simulink model "ESS_3P_2L_220kW_for_LS_Project"  (R2023b)
settings: Solver=VariableStepAuto  StartTime=0.0  StopTime=3  RelTol=1e-3
InitFcn:
  | %Initialization_for_ESS_3P_2L_220kW;
  | Initialization_for_ESS_3P_2L_220kW;
values from neighbouring files (symbols this model uses):
  C_grid = 54e-6    (= 5.4e-05)    [Initialization_for_ESS_3P_2L_220kW.m]    (also in Initialization_for_Testbench.m = 4.5e-05)
  Cdc = 180e-6    (= 0.00018)    [CurrentLoop.m]    (also in Initialization_for_ESS_3P_2L_220kW.m; Initialization_for_Testbench.m)
  Fnom_Grid = 50    [CurrentLoop.m]    (also in Initialization_for_ESS_3P_2L_220kW.m; Initialization_for_Testbench.m)
  Gain_for_ActiveDamping = 1    [Initialization_for_Testbench.m]
  Inom = Pnom/sqrt(3)/Unom_Grid    [CurrentLoop.m]    (also in Initialization_for_ESS_3P_2L_220kW.m; Initialization_for_Testbench.m)
  Ki_Edq = Kp_Edq*2*pi*10    (= 18.8495559215)    [Initialization_for_ESS_3P_2L_220kW.m]
  Ki_Idq = Kp_Idq*2*pi*10    (= 157.913670417)    [Initialization_for_ESS_3P_2L_220kW.m]    (also in Initialization_for_Testbench.m = 1.26330936334)
  Kp_Edq = 0.3    [Initialization_for_ESS_3P_2L_220kW.m]
  Kp_Idq = L_grid*2*pi*2000    (= 2.51327412287)    [Initialization_for_ESS_3P_2L_220kW.m]    (also in Initialization_for_Testbench.m = 2.0106192983)
  L_grid = 200e-6    (= 0.0002)    [Initialization_for_ESS_3P_2L_220kW.m]    (also in Initialization_for_Testbench.m)
  Pnom = 220e3    (= 220000)    [CurrentLoop.m]    (also in Initialization_for_ESS_3P_2L_220kW.m; Initialization_for_Testbench.m = 2500000)
  Ts_Control = 62.5e-6    (= 6.25e-05)    [CurrentLoop.m]    (also in Initialization_for_ESS_3P_2L_220kW.m; Initialization_for_Testbench.m = 0.0001)
  Ts_Power = 10e-7    (= 1e-06)    [Initialization_for_ESS_3P_2L_220kW.m]    (also in Initialization_for_Testbench.m)
  Udc_ref = 1500    [CurrentLoop.m]    (also in Initialization_for_ESS_3P_2L_220kW.m; Initialization_for_Testbench.m)
  Unom_Grid = 690    [CurrentLoop.m]    (also in Initialization_for_ESS_3P_2L_220kW.m; Initialization_for_Testbench.m)
  Unom_Phase = Unom_Grid/sqrt(3)    [CurrentLoop.m]    (also in Initialization_for_ESS_3P_2L_220kW.m; Initialization_for_Testbench.m)
undefined symbols (not defined in the file or in its folder): DiscIntNeverNeededParam, magnitude
libraries: LibraryForCodeGeneration x15, slpidlib x10, spsabctodq0Lib x7, spsAlphaBetaZerotoabcLib x6, simulink x5, spsThreePhaseVIMeasurementLib x4, spsVoltageMeasurementLib x4, eeGeneralControl x3, spsabctoAlphaBetaZeroLib x3, spsSeriesRLCBranchLib x3, spsThreePhaseSeriesRLCBranchLib x3, spsStairGeneratorLib x2
(part 2 of 2)

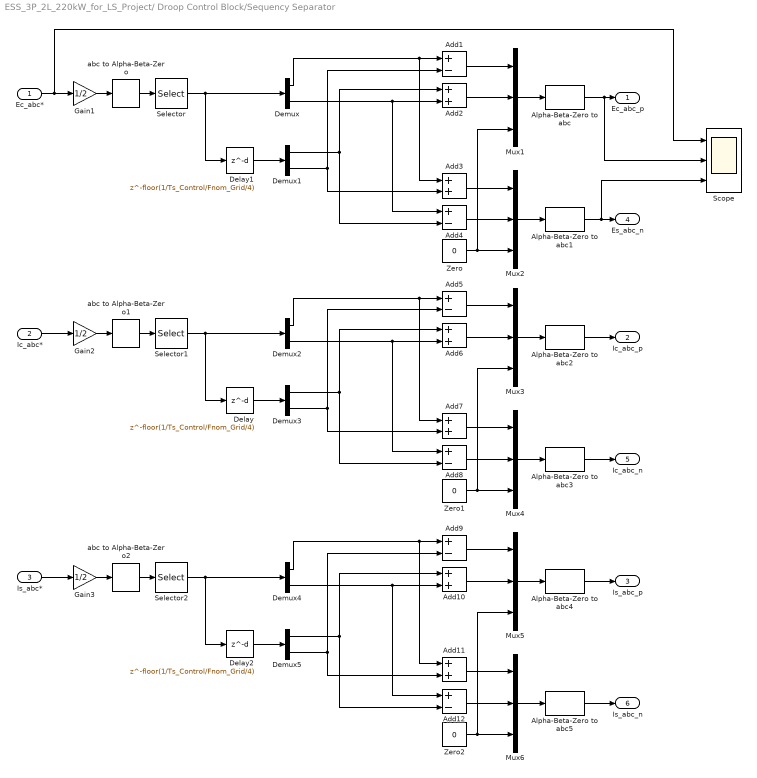
== system ESS_3P_2L_220kW_for_LS_Project/ Droop Control Block/Sequency Separator ==
  Ec_abc* : Inport
  " Ic_abc*" : Inport  Port=2
  Is_abc* : Inport  Port=3
  Add{1,4..5,8..9,12} (6 alike) : Sum  Inputs=+-
  Add{2..3,6..7,10..11} (6 alike) : Sum
  Alpha-Beta-Zero to abc{,1..5} (6 alike) : spsAlphaBetaZerotoabcLib/Alpha-Beta-Zero to abc
  Delay : Delay  DelayLength=floor(1/Ts_Control/Fnom_Grid/4)  SampleTime=Ts_Control
  Delay1 : Delay  DelayLength=floor(1/Ts_Control/Fnom_Grid/4)  SampleTime=Ts_Control
  Delay2 : Delay  DelayLength=floor(1/Ts_Control/Fnom_Grid/4)  SampleTime=Ts_Control
  Demux{,1..5} (6 alike) : Demux  Outputs=2
  Gain1 : Gain  Gain=1/2
  Gain2 : Gain  Gain=1/2
  Gain3 : Gain  Gain=1/2
  Mux{1..6} (6 alike) : Mux  Inputs=3
  Scope : Scope  NumInputPorts=3
  Selector : Selector  InputPortWidth=3  IndexOptions=Index vector (dialog)  Indices=[1 2]  OutputSizes=1
  Selector1 : Selector  InputPortWidth=3  IndexOptions=Index vector (dialog)  Indices=[1 2]  OutputSizes=1
  Selector2 : Selector  InputPortWidth=3  IndexOptions=Index vector (dialog)  Indices=[1 2]  OutputSizes=1
  Zero : Constant  Value=0  OutDataTypeStr=Inherit: Inherit via back propagation
  Zero1 : Constant  Value=0  OutDataTypeStr=Inherit: Inherit via back propagation
  Zero2 : Constant  Value=0  OutDataTypeStr=Inherit: Inherit via back propagation
  abc to Alpha-Beta-Zero : spsabctoAlphaBetaZeroLib/abc to Alpha-Beta-Zero
  abc to Alpha-Beta-Zero1 : spsabctoAlphaBetaZeroLib/abc to Alpha-Beta-Zero
  abc to Alpha-Beta-Zero2 : spsabctoAlphaBetaZeroLib/abc to Alpha-Beta-Zero
  Ec_abc_p : Outport
  Ic_abc_p : Outport  Port=2
  Is_abc_p : Outport  Port=3
  Es_abc_n : Outport  Port=4
  Ic_abc_n : Outport  Port=5
  Is_abc_n : Outport  Port=6
  wires:
  Is_abc*/1 -> Gain3/1
  Demux4/2 -> Add10/2, Add12/1
  Demux5/1 -> Add10/1, Add12/2
  Demux5/2 -> Add9/2, Add11/2
  Gain3/1 -> abc to Alpha-Beta-Zero2/1
  Demux4/1 -> Add9/1, Add11/1
  Delay2/1 -> Demux5/1
  Add12/1 -> Mux6/2
  Add11/1 -> Mux6/1
  Add10/1 -> Mux5/2
  Add9/1 -> Mux5/1
  Alpha-Beta-Zero to abc5/1 -> Is_abc_n/1
  Alpha-Beta-Zero to abc4/1 -> Is_abc_p/1
  Zero2/1 -> Mux6/3, Mux5/3
  Selector2/1 -> Demux4/1, Delay2/1
  abc to Alpha-Beta-Zero2/1 -> Selector2/1
  Mux5/1 -> Alpha-Beta-Zero to abc4/1
  Mux6/1 -> Alpha-Beta-Zero to abc5/1
  " Ic_abc*"/1 -> Gain2/1
  Mux4/1 -> Alpha-Beta-Zero to abc3/1
  Mux3/1 -> Alpha-Beta-Zero to abc2/1
  abc to Alpha-Beta-Zero1/1 -> Selector1/1
  Selector1/1 -> Delay/1, Demux2/1
  Zero1/1 -> Mux3/3, Mux4/3
  Alpha-Beta-Zero to abc2/1 -> Ic_abc_p/1
  Alpha-Beta-Zero to abc3/1 -> Ic_abc_n/1
  Add5/1 -> Mux3/1
  Add6/1 -> Mux3/2
  Add7/1 -> Mux4/1
  Add8/1 -> Mux4/2
  Delay/1 -> Demux3/1
  Demux2/1 -> Add7/1, Add5/1
  Gain2/1 -> abc to Alpha-Beta-Zero1/1
  Demux3/2 -> Add7/2, Add5/2
  Demux3/1 -> Add8/2, Add6/1
  Demux2/2 -> Add8/1, Add6/2
  Demux/2 -> Add2/2, Add4/1
  Demux1/1 -> Add2/1, Add4/2
  Demux1/2 -> Add1/2, Add3/2
  Gain1/1 -> abc to Alpha-Beta-Zero/1
  Demux/1 -> Add1/1, Add3/1
  Delay1/1 -> Demux1/1
  Add4/1 -> Mux2/2
  Add3/1 -> Mux2/1
  Add2/1 -> Mux1/2
  Add1/1 -> Mux1/1
  Alpha-Beta-Zero to abc1/1 -> Es_abc_n/1, Scope/3
  Alpha-Beta-Zero to abc/1 -> Ec_abc_p/1, Scope/2
  Zero/1 -> Mux2/3, Mux1/3
  Selector/1 -> Demux/1, Delay1/1
  abc to Alpha-Beta-Zero/1 -> Selector/1
  Mux1/1 -> Alpha-Beta-Zero to abc/1
  Mux2/1 -> Alpha-Beta-Zero to abc1/1
  Ec_abc*/1 -> Scope/1, Gain1/1

== system ESS_3P_2L_220kW_for_LS_Project/ Droop Control Block/Synchronous Phase ==
  Ec_abc : Inport
  Egrid_abc : Inport  Port=2
  En_SP : Inport  Port=3
  AND : Logic  IconShape=distinctive  AllPortsSameDT=off  OutDataTypeStr=boolean
  Abs : Abs  SaturateOnIntegerOverflow=off
  Abs1 : Abs  SaturateOnIntegerOverflow=off
  Compare To Constant : simulink/Logic and Bit Operations/Compare To Constant  relop=<=  const=3  OutDataTypeStr=boolean
  Compare To Constant1 : simulink/Logic and Bit Operations/Compare To Constant  relop=<=  const=100e-3  OutDataTypeStr=boolean
  Constant : Constant  Value=[0,0]
  Demux : Demux  Outputs=2
  Index Vector : MultiPortSwitch  DataPortOrder=Zero-based contiguous  Inputs=2  zeroidx=on  SaturateOnIntegerOverflow=off  InputSameDT=off
  Moving Average : eeGeneralControl/Moving Average  VariantControl=Variant1  LabelModeActiveChoice=Discrete  f=0.1*Fnom_Grid  x0=0  BufferSize=8192  Ts=Ts_Control
      settings: LibrarySourceBlock=ee_sl_lib/General Control/Moving Average
  Moving Average1 : eeGeneralControl/Moving Average  VariantControl=Variant1  LabelModeActiveChoice=Discrete  f=0.1*Fnom_Grid  x0=0  BufferSize=8192  Ts=Ts_Control
      settings: LibrarySourceBlock=ee_sl_lib/General Control/Moving Average
  Subsystem : Subsystem
  COM : Outport
  Delta_Es : Outport  Port=2
  wires:
  Moving Average/1 -> Compare To Constant/1
  Abs/1 -> Moving Average/1
  Moving Average1/1 -> Compare To Constant1/1
  Abs1/1 -> Moving Average1/1
  AND/1 -> COM/1
  Compare To Constant/1 -> AND/1
  Compare To Constant1/1 -> AND/2
  Subsystem/1(Delta_Es) -> Demux/1, Index Vector/3
  Egrid_abc/1 -> Subsystem/1(Es)
  Ec_abc/1 -> Subsystem/2(Ec)
  En_SP/1 -> Subsystem/Enable, Index Vector/1
  Demux/1 -> Abs/1
  Demux/2 -> Abs1/1
  Index Vector/1 -> Delta_Es/1
  Constant/1 -> Index Vector/2

== system ESS_3P_2L_220kW_for_LS_Project/ Droop Control Block/Udq2Uabc ==
  Udq_p : Inport
  Udq_n : Inport  Port=2
  wt : Inport  Port=3
  Add : Sum
  Gain2 : Gain  Gain=-1
  Mux1 : Mux  Inputs=2
  Mux2 : Mux  Inputs=2
  Saturation : Saturate  UpperLimit=1.15  LowerLimit=-1.15
  Scope : Scope  NumInputPorts=3
  Zero1 : Constant  Value=0  OutDataTypeStr=Inherit: Inherit via back propagation
  Zero2 : Constant  Value=0  OutDataTypeStr=Inherit: Inherit via back propagation
  dq0 to abc : spsdq0toabcLib/dq0 to abc  Alignment=Aligned with phase A axis
  dq0 to abc1 : spsdq0toabcLib/dq0 to abc  Alignment=Aligned with phase A axis
  Uabc : Outport
  wires:
  Saturation/1 -> Uabc/1
  Zero2/1 -> Mux1/2
  dq0 to abc/1 -> Add/1, Scope/1
  Add/1 -> Scope/3, Saturation/1
  Udq_n/1 -> Mux2/1
  Mux2/1 -> dq0 to abc1/1
  Udq_p/1 -> Mux1/1
  Mux1/1 -> dq0 to abc/1
  Zero1/1 -> Mux2/2
  Gain2/1 -> dq0 to abc1/2
  wt/1 -> dq0 to abc/2, Gain2/1
  dq0 to abc1/1 -> Add/2, Scope/2

== system ESS_3P_2L_220kW_for_LS_Project/ Droop Control Block/Voltage Conversion ==
  Phase-Phase : Inport
  Add : Sum  Inputs=+-
  Add1 : Sum
  Add2 : Sum  Inputs=--
  Demux : Demux  Outputs=3
  Gain : Gain  Gain=1/3
  Gain1 : Gain  Gain=2
  Gain2 : Gain  Gain=2
  Mux : Mux  Inputs=3
  Terminator : Terminator
  Phase-Ground : Outport
  wires:
  Demux/3 -> Terminator/1
  Gain2/1 -> Add2/2
  Gain1/1 -> Add1/1
  Demux/2 -> Add/1, Add1/2, Gain2/1
  Demux/1 -> Gain1/1, Add2/1, Add/2
  Add2/1 -> Mux/3
  Add1/1 -> Mux/1
  Add/1 -> Mux/2
  Mux/1 -> Phase-Ground/1
  Gain/1 -> Demux/1
  Phase-Phase/1 -> Gain/1

== system ESS_3P_2L_220kW_for_LS_Project/ Droop Control Block/Voltage Conversion1 ==
  Phase-Phase : Inport
  Add : Sum  Inputs=+-
  Add1 : Sum
  Add2 : Sum  Inputs=--
  Demux : Demux  Outputs=3
  Gain : Gain  Gain=1/3
  Gain1 : Gain  Gain=2
  Gain2 : Gain  Gain=2
  Mux : Mux  Inputs=3
  Terminator : Terminator
  Phase-Ground : Outport
  wires:
  Demux/3 -> Terminator/1
  Gain2/1 -> Add2/2
  Gain1/1 -> Add1/1
  Demux/2 -> Add/1, Add1/2, Gain2/1
  Demux/1 -> Gain1/1, Add2/1, Add/2
  Add2/1 -> Mux/3
  Add1/1 -> Mux/1
  Add/1 -> Mux/2
  Mux/1 -> Phase-Ground/1
  Gain/1 -> Demux/1
  Phase-Phase/1 -> Gain/1

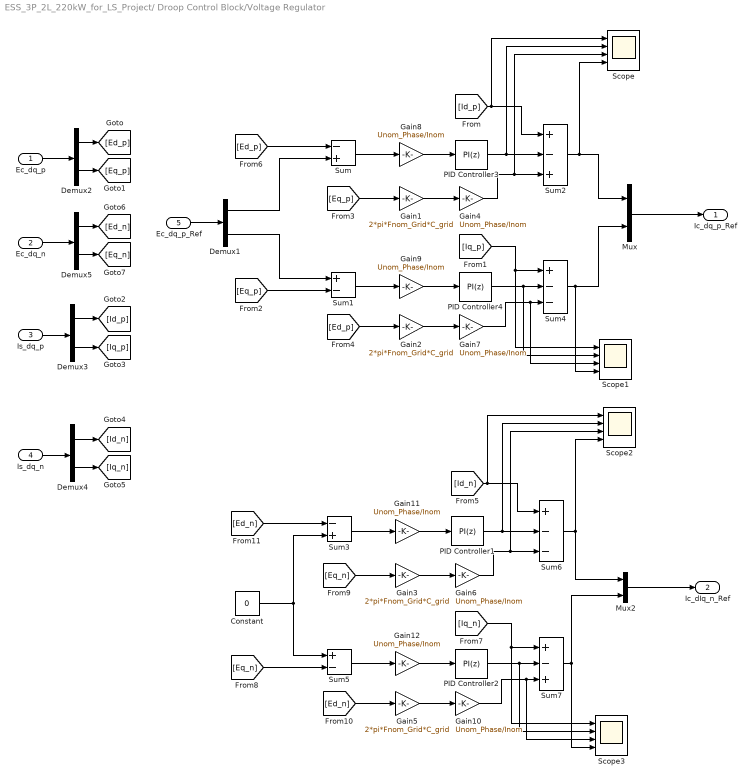
== system ESS_3P_2L_220kW_for_LS_Project/ Droop Control Block/Voltage Regulator ==
  Ec_dq_p : Inport
  Ec_dq_n : Inport  Port=2
  Is_dq_p : Inport  Port=3
  Is_dq_n : Inport  Port=4
  Ec_dq_p_Ref : Inport  Port=5  PortDimensions=2
  Constant : Constant  Value=0
  Demux{1..5} (5 alike) : Demux  Outputs=2
  Gain{1..3,5} (4 alike) : Gain  Gain=2*pi*Fnom_Grid*C_grid
  Gain{4,6..12} (8 alike) : Gain  Gain=Unom_Phase/Inom
  Mux : Mux  Inputs=2
  Mux2 : Mux  Inputs=2
  PID Controller{1..4} (4 alike) : slpidlib/PID Controller  Controller=PI  Form=Parallel  TimeDomain=Discrete-time  UseExternalTs=off  SampleTime=Ts_Control  IntegratorMethod=Forward Euler  FilterMethod=Forward Euler  ControllerParametersSource=internal  P=Kp_Edq  I=Ki_Edq  UseKiTs=off  D=0  N=100  UseFilter=on  TunerSelectOption=Transfer Function Based (PID Tuner App)  InitialConditionSource=internal  InitialConditionForIntegrator=0  InitialConditionForFilter=0  DifferentiatorICPrevScaledInput=0  ExternalReset=none  TrackingMode=off  Kt=1  LimitOutput=on  SatLimitsSource=internal  UpperSaturationLimit=2  LowerSaturationLimit=-2  LinearizeAsGain=on  AntiWindupMode=clamping  Kb=1  LimitIntegrator=off  UpperIntegratorSaturationLimit=inf  LowerIntegratorSaturationLimit=-inf  POutMin=[]  POutMax=[]  IOutMin=[]  IOutMax=[]  DOutMin=[]  DOutMax=[]  NOutMin=[]  NOutMax=[]  SumOutMin=[]  SumOutMax=[]  SaturationOutMin=[]  SaturationOutMax=[]  PParamMin=[]  PParamMax=[]  IParamMin=[]  IParamMax=[]  DParamMin=[]  DParamMax=[]  NParamMin=[]  NParamMax=[]  KbParamMin=[]  KbParamMax=[]  KtParamMin=[]  KtParamMax=[]  KbOutMin=[]  KbOutMax=[]  KtOutMin=[]  KtOutMax=[]  IntegratorOutMin=[]  IntegratorOutMax=[]  FilterOutMin=[]  FilterOutMax=[]  SumI1OutMin=[]  SumI1OutMax=[]  SumI2OutMin=[]  SumI2OutMax=[]  SumI3OutMin=[]  SumI3OutMax=[]  SumI4OutMin=[]  SumI4OutMax=[]  SumDOutMin=[]  SumDOutMax=[]  DifferentiatorOutMin=[]  DifferentiatorOutMax=[]  FilterDiffOutCoefMin=[]  FilterDiffOutCoefMax=[]  ReciprocalOutMin=[]  ReciprocalOutMax=[]  SumDenOutMin=[]  SumDenOutMax=[]  SumNumOutMin=[]  SumNumOutMax=[]  DivideOutMin=[]  DivideOutMax=[]  UdiffTsProdOutMin=[]  UdiffTsProdOutMax=[]  NTsProdOutMin=[]  NTsProdOutMax=[]  UintegralTsProdOutMin=[]  UintegralTsProdOutMax=[]  UngainTsProdOutMin=[]  UngainTsProdOutMax=[]  ClampingZeroOutDataTypeStr=Inherit: Inherit via back propagation  ClampingZeroOutMin=[]  ClampingZeroOutMax=[]  FilterDenConstantOutDataTypeStr=Inherit: Inherit via back propagation  FilterDenConstantOutMin=[]  FilterDenConstantOutMax=[]  PCopyOutDataTypeStr=Inherit: Inherit via back propagation  PCopyOutMin=[]  PCopyOutMax=[]  NCopyOutDataTypeStr=Inherit: Inherit via back propagation  NCopyOutMin=[]  NCopyOutMax=[]  IntegratorContinuousStateAttributes=''  IntegratorStateMustResolveToSignalObject=off  IntegratorRTWStateStorageClass=Auto  FilterContinuousStateAttributes=''  FilterStateMustResolveToSignalObject=off  FilterRTWStateStorageClass=Auto  ParallelPVariant=InternalParameters  IdealPVariant=Disabled  IVariant=InternalParameters  DVariant=Disabled  IntegratorVariant=Discrete  SatVariant=Enabled  AWVariant=DiscClampingParallel  PCopyVariant=Disabled  TRVariant=Disabled  FdbkBlocksVariant=Forward  IdealPFdbkVariant=Disabled  SatFdbkVariant=Disabled  DerivativeFilterVariant=Disabled  NVariant=Disabled  NCopyVariant=Disabled_SignalSpec  FilterICVariant=Disabled  IntegratorICVariant=InternalICs  ExternalResetVariant=Disabled  TRSumVariant=Passthrough  SumFdbkVariant=Disabled  SumVariant=Sum_PI  TsampFilterVariant=InternalTs  TsampNgainVariant=Passthrough  TsampIntegralVariant=Disabled_SignalSpec  ExternalSaturationOutDataTypeStr=Inherit: Same as second input
  Scope{,1..3} (4 alike) : Scope  NumInputPorts=4
  Sum : Sum  Inputs=-+  InputSameDT=on  SaturateOnIntegerOverflow=on  OutDataTypeStr=Inherit: Same as first input
  Sum1 : Sum  Inputs=+-  InputSameDT=on  SaturateOnIntegerOverflow=on  OutDataTypeStr=Inherit: Same as first input
  Sum2 : Sum  Inputs=+-+  InputSameDT=on  SaturateOnIntegerOverflow=on  OutDataTypeStr=Inherit: Same as first input
  Sum3 : Sum  Inputs=-+  InputSameDT=on  SaturateOnIntegerOverflow=on  OutDataTypeStr=Inherit: Same as first input
  Sum4 : Sum  Inputs=+--  InputSameDT=on  SaturateOnIntegerOverflow=on  OutDataTypeStr=Inherit: Same as first input
  Sum5 : Sum  Inputs=+-  InputSameDT=on  SaturateOnIntegerOverflow=on  OutDataTypeStr=Inherit: Same as first input
  Sum6 : Sum  Inputs=+--  InputSameDT=on  SaturateOnIntegerOverflow=on  OutDataTypeStr=Inherit: Same as first input
  Sum7 : Sum  Inputs=+-+  InputSameDT=on  SaturateOnIntegerOverflow=on  OutDataTypeStr=Inherit: Same as first input
  Ic_dq_p_Ref : Outport
  Ic_dIq_n_Ref : Outport  Port=2
  wires:
  Demux2/1 -> [Ed_p]
  [Ed_p] -> Gain2/1
  [Ed_p] -> Sum/1
  Sum2/1 -> Scope/4, Mux/1
  Gain8/1 -> PID Controller3/1
  Is_dq_p/1 -> Demux3/1
  Demux1/1 -> Sum/2
  Demux3/2 -> [Iq_p]
  Gain4/1 -> Scope/3, Sum2/3
  Demux1/2 -> Sum1/1
  Demux3/1 -> [Id_p]
  Sum4/1 -> Scope1/4, Mux/2
  [Eq_p] -> Sum1/2
  [Iq_p] -> Sum4/1, Scope1/1
  [Eq_p] -> Gain1/1
  Ec_dq_p/1 -> Demux2/1
  Sum1/1 -> Gain9/1
  Sum/1 -> Gain8/1
  Ec_dq_p_Ref/1 -> Demux1/1
  Gain1/1 -> Gain4/1
  Gain9/1 -> PID Controller4/1
  Gain7/1 -> Scope1/3, Sum4/3
  Gain2/1 -> Gain7/1
  PID Controller4/1 -> Scope1/2, Sum4/2
  PID Controller3/1 -> Scope/2, Sum2/2
  Demux2/2 -> [Eq_p]
  [Id_p] -> Scope/1, Sum2/1
  Mux/1 -> Ic_dq_p_Ref/1
  Demux4/2 -> [Iq_n]
  Demux4/1 -> [Id_n]
  Is_dq_n/1 -> Demux4/1
  Gain5/1 -> Gain10/1
  [Id_n] -> Scope2/1, Sum6/1
  PID Controller1/1 -> Scope2/2, Sum6/2
  PID Controller2/1 -> Scope3/2, Sum7/2
  Gain11/1 -> PID Controller1/1
  Sum3/1 -> Gain11/1
  Sum6/1 -> Mux2/1, Scope2/4
  Gain10/1 -> Scope3/3, Sum7/3
  [Iq_n] -> Sum7/1, Scope3/1
  Gain3/1 -> Gain6/1
  [Eq_n] -> Gain3/1
  [Eq_n] -> Sum5/2
  Sum5/1 -> Gain12/1
  Sum7/1 -> Mux2/2, Scope3/4
  Gain6/1 -> Scope2/3, Sum6/3
  [Ed_n] -> Sum3/1
  Gain12/1 -> PID Controller2/1
  [Ed_n] -> Gain5/1
  Constant/1 -> Sum5/1, Sum3/2
  Demux5/2 -> [Eq_n]
  Ec_dq_n/1 -> Demux5/1
  Demux5/1 -> [Ed_n]
  Mux2/1 -> Ic_dIq_n_Ref/1

== system ESS_3P_2L_220kW_for_LS_Project/ Droop Control Block/abc2dq_n ==
  Ec_abc_n : Inport
  "Ic_abc_n " : Inport  Port=2
  Is_abc_n : Inport  Port=3
  wt : Inport  Port=4
  Gain2 : Gain  Gain=-1
  Selector : Selector  InputPortWidth=3  IndexOptions=Index vector (dialog)  Indices=[1 2]  OutputSizes=1
  Selector1 : Selector  InputPortWidth=3  IndexOptions=Index vector (dialog)  Indices=[1 2]  OutputSizes=1
  Selector2 : Selector  InputPortWidth=3  IndexOptions=Index vector (dialog)  Indices=[1 2]  OutputSizes=1
  abc to dq0 : spsabctodq0Lib/abc to dq0  Alignment=Aligned with phase A axis
  abc to dq1 : spsabctodq0Lib/abc to dq0  Alignment=Aligned with phase A axis
  abc to dq2 : spsabctodq0Lib/abc to dq0  Alignment=Aligned with phase A axis
  Ec_dq_n : Outport
  Ic_dq_n : Outport  Port=2
  Is_dq_n : Outport  Port=3
  wires:
  Gain2/1 -> abc to dq0/2, abc to dq1/2, abc to dq2/2
  Is_abc_n/1 -> abc to dq2/1
  abc to dq2/1 -> Selector2/1
  Selector2/1 -> Is_dq_n/1
  wt/1 -> Gain2/1
  Ec_abc_n/1 -> abc to dq0/1
  "Ic_abc_n "/1 -> abc to dq1/1
  abc to dq1/1 -> Selector1/1
  abc to dq0/1 -> Selector/1
  Selector/1 -> Ec_dq_n/1
  Selector1/1 -> Ic_dq_n/1

== system ESS_3P_2L_220kW_for_LS_Project/ Droop Control Block/abc2dq_p ==
  Ec_abc_p : Inport
  "Ic_abc_p " : Inport  Port=2
  Is_abc_p : Inport  Port=3
  wt : Inport  Port=4
  Selector : Selector  InputPortWidth=3  IndexOptions=Index vector (dialog)  Indices=[1 2]  OutputSizes=1
  Selector1 : Selector  InputPortWidth=3  IndexOptions=Index vector (dialog)  Indices=[1 2]  OutputSizes=1
  Selector2 : Selector  InputPortWidth=3  IndexOptions=Index vector (dialog)  Indices=[1 2]  OutputSizes=1
  abc to dq0 : spsabctodq0Lib/abc to dq0  Alignment=Aligned with phase A axis
  abc to dq1 : spsabctodq0Lib/abc to dq0  Alignment=Aligned with phase A axis
  abc to dq2 : spsabctodq0Lib/abc to dq0  Alignment=Aligned with phase A axis
  Ec_dq_p : Outport
  Ic_dq_p : Outport  Port=2
  Is_dq_p : Outport  Port=3
  wires:
  abc to dq2/1 -> Selector2/1
  Selector2/1 -> Is_dq_p/1
  Is_abc_p/1 -> abc to dq2/1
  wt/1 -> abc to dq0/2, abc to dq1/2, abc to dq2/2
  Selector1/1 -> Ic_dq_p/1
  Selector/1 -> Ec_dq_p/1
  abc to dq0/1 -> Selector/1
  abc to dq1/1 -> Selector1/1
  "Ic_abc_p "/1 -> abc to dq1/1
  Ec_abc_p/1 -> abc to dq0/1

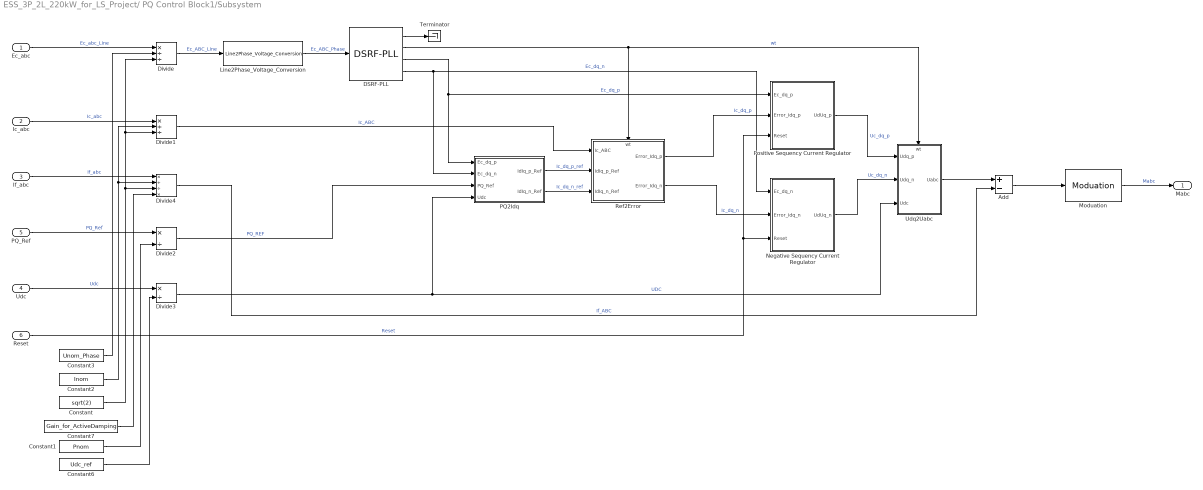
== system ESS_3P_2L_220kW_for_LS_Project/ PQ Control Block1/Subsystem ==
  Ec_abc : Inport  OutDataTypeStr=single  PortDimensions=3
  Ic_abc : Inport  Port=2  OutDataTypeStr=single  PortDimensions=3
  If_abc : Inport  Port=3  OutDataTypeStr=single  PortDimensions=3
  Udc : Inport  Port=4  OutDataTypeStr=single
  PQ_Ref : Inport  Port=5  OutDataTypeStr=single
  Reset : Inport  Port=6  OutDataTypeStr=boolean
  Add : Sum  Inputs=+-
  Constant : Constant  Value=sqrt(2)  OutDataTypeStr=Inherit: Inherit via back propagation  SampleTime=-1
  Constant1 : Constant  Value=Pnom  OutDataTypeStr=Inherit: Inherit via back propagation  SampleTime=-1
  Constant2 : Constant  Value=Inom  OutDataTypeStr=Inherit: Inherit via back propagation  SampleTime=-1
  Constant3 : Constant  Value=Unom_Phase  OutDataTypeStr=Inherit: Inherit via back propagation  SampleTime=-1
  Constant6 : Constant  Value=Udc_ref  OutDataTypeStr=Inherit: Inherit via back propagation  SampleTime=-1
  Constant7 : Constant  Value=Gain_for_ActiveDamping  OutDataTypeStr=Inherit: Inherit via back propagation  SampleTime=-1
  DSRF-PLL : LibraryForCodeGeneration/DSRF-PLL  Ts=Ts_Control  Wc=2*pi*50*0.707  Wf=2*pi*50  Kp=2*pi*25*2*0.707  Ki=power(2*pi*25,2)
  Divide : Product  Inputs=*//  OutDataTypeStr=single
  Divide1 : Product  Inputs=*//  OutDataTypeStr=single
  Divide2 : Product  Inputs=*/  OutDataTypeStr=single
  Divide3 : Product  Inputs=*/  OutDataTypeStr=single
  Divide4 : Product  Inputs=*//*  OutDataTypeStr=single
  Line2Phase_Voltage_Conversion : LibraryForCodeGeneration/Line2Phase_Voltage_Conversion  SystemSampleTime=-1  VariantActivationTime=update diagram  AllowFlexibleInterface=on  Latency=0  AutoFrameSizeCalculation=off
  Moduation : LibraryForCodeGeneration/Moduation  Modulation=SPWM
  Negative Sequency Current Regulator : Subsystem
  PQ2Idq : Subsystem  TreatAsAtomicUnit=on
  Positive Sequency Current Regulator : Subsystem
  Ref2Error : Subsystem
      settings: PortSchema="{\"entries\":[{\"content\":{\"sides\":[{\"content\":{\"connectorIds\":[\"In1\",\"In2\",\"In3\"]},\"type\":\"ConnectorPlacement.EquallySpacedRectSide\",\"uuid\":\"702c7fae-dbbb-427d-af19-afd468018ae6\"},{\"content\":{\"connectorIds\":[\"Out1\",\"Out2\"],\"side\":\"RIGHT\"},\"type\":\"ConnectorPlacement.EquallySpacedRectSide\",\"uuid\":\"d2ca5462-a446-46d8-bb73-1a455ffa959f\"},{\"content\":{\"connectorIds\":[\"In4\"],\"side\":\"TOP\"},\"type\":\"ConnectorPlacement.EquallySpacedRectSide\",\"uuid\":\"50bc6c44-424f-4342-960e-11540364fe97\"}]},\"type\":\"ConnectorPlacement.EquallySpacedConnector\",\"uuid\":\"f58cf64d-fe35-43f1-a031-7ee625a8bb1e\"}],\"packageUris\":[\"http://schema.mathworks.com/mf0/Connector/R2020b\"],\"version\":\"1.0\"}"
  Terminator : Terminator
  Udq2Uabc : Subsystem
      settings: PortSchema="{\"entries\":[{\"content\":{\"sides\":[{\"content\":{\"connectorIds\":[\"In1\",\"In2\",\"In3\"]},\"type\":\"ConnectorPlacement.EquallySpacedRectSide\",\"uuid\":\"009786f4-728c-4160-b9bf-eaf0b5a05101\"},{\"content\":{\"connectorIds\":[\"Out1\"],\"side\":\"RIGHT\"},\"type\":\"ConnectorPlacement.EquallySpacedRectSide\",\"uuid\":\"2a94367a-5c57-4632-9573-ab089470159a\"},{\"content\":{\"connectorIds\":[\"In4\"],\"side\":\"TOP\"},\"type\":\"ConnectorPlacement.EquallySpacedRectSide\",\"uuid\":\"6906365b-3187-4c4b-97cf-c9dec4c5ef7c\"}]},\"type\":\"ConnectorPlacement.EquallySpacedConnector\",\"uuid\":\"96ca8566-a266-405c-817a-b47b433d51ed\"}],\"packageUris\":[\"http://schema.mathworks.com/mf0/Connector/R2020b\"],\"version\":\"1.0\"}"
  Mabc : Outport  OutDataTypeStr=single  PortDimensions=3
  wires:
  Constant1/1 -> Divide2/2
  Negative Sequency Current Regulator/1(UdUq_n) -> Udq2Uabc/2(Udq_n)  "Uc_dq_n"
  Divide4/1 -> Add/2  "If_ABC"
  Udq2Uabc/1(Uabc) -> Add/1
  Constant6/1 -> Divide3/2
  Constant7/1 -> Divide4/4
  PQ_Ref/1 -> Divide2/1  "PQ_Ref"
  Add/1 -> Moduation/1
  DSRF-PLL/1 -> Terminator/1
  Moduation/1 -> Mabc/1  "Mabc"
  Reset/1 -> Positive Sequency Current Regulator/3(Reset), Negative Sequency Current Regulator/3(Reset)  "Reset"
  DSRF-PLL/2 -> Udq2Uabc/4(wt), Ref2Error/4(wt)  "wt"
  If_abc/1 -> Divide4/1  "If_abc"
  DSRF-PLL/4 -> PQ2Idq/2(Ec_dq_n), Negative Sequency Current Regulator/1(Ec_dq_n)  "Ec_dq_n"
  PQ2Idq/2(IdIq_n_Ref) -> Ref2Error/3(IdIq_n_Ref)  "Ic_dq_n_ref"
  Divide/1 -> Line2Phase_Voltage_Conversion/1  "Ec_ABC_Line"
  Udc/1 -> Divide3/1  "Udc"
  Constant/1 -> Divide4/3, Divide1/3, Divide/3
  Constant3/1 -> Divide/2
  Divide1/1 -> Ref2Error/1("Ic_ABC ")  "Ic_ABC"
  DSRF-PLL/3 -> Positive Sequency Current Regulator/1(Ec_dq_p), PQ2Idq/1(Ec_dq_p)  "Ec_dq_p"
  PQ2Idq/1(IdIq_p_Ref) -> Ref2Error/2("IdIq_p_Ref ")  "Ic_dq_p_ref"
  Positive Sequency Current Regulator/1(UdUq_p) -> Udq2Uabc/1(Udq_p)  "Uc_dq_p"
  Ref2Error/2(Error_Idq_n) -> Negative Sequency Current Regulator/2(Error_Idq_n)  "Ic_dq_n"
  Divide3/1 -> Udq2Uabc/3(Udc), PQ2Idq/4(Udc)  "UDC"
  Divide2/1 -> PQ2Idq/3(PQ_Ref)  "PQ_REF"
  Ic_abc/1 -> Divide1/1  "Ic_abc"
  Constant2/1 -> Divide4/2, Divide1/2
  Ref2Error/1(Error_Idq_p) -> Positive Sequency Current Regulator/2(Error_Idq_p)  "Ic_dq_p"
  Line2Phase_Voltage_Conversion/1 -> DSRF-PLL/1  "Ec_ABC_Phase"
  Ec_abc/1 -> Divide/1  "Ec_abc_Line"

== system ESS_3P_2L_220kW_for_LS_Project/ Droop Control Block/Synchronous Phase/Subsystem ==
  Es : Inport
  Ec : Inport  Port=2
  Enable : EnablePort  StatesWhenEnabling=reset
  Add1 : Sum  Inputs=-+
  Add2 : Sum  Inputs=+-
  Add3 : Sum  Inputs=-+
  Constant1 : Constant  Value=0
  Constant2 : Constant  Value=pi/2
  Constant3 : Constant
  Mux : Mux  Inputs=2
  PID Controller1 : slpidlib/PID Controller  Controller=PI  Form=Parallel  TimeDomain=Discrete-time  UseExternalTs=off  SampleTime=Ts_Control  IntegratorMethod=Forward Euler  FilterMethod=Forward Euler  ControllerParametersSource=internal  P=Kp_Edq*1  I=Kp_Edq*2*pi*0.01  UseKiTs=off  D=0  N=100  UseFilter=on  TunerSelectOption=Transfer Function Based (PID Tuner App)  InitialConditionSource=internal  InitialConditionForIntegrator=0  InitialConditionForFilter=0  DifferentiatorICPrevScaledInput=0  ExternalReset=none  TrackingMode=off  Kt=1  LimitOutput=on  SatLimitsSource=internal  UpperSaturationLimit=0.2  LowerSaturationLimit=-0.2  LinearizeAsGain=on  AntiWindupMode=clamping  Kb=1  LimitIntegrator=off  UpperIntegratorSaturationLimit=inf  LowerIntegratorSaturationLimit=-inf  POutMin=[]  POutMax=[]  IOutMin=[]  IOutMax=[]  DOutMin=[]  DOutMax=[]  NOutMin=[]  NOutMax=[]  SumOutMin=[]  SumOutMax=[]  SaturationOutMin=[]  SaturationOutMax=[]  PParamMin=[]  PParamMax=[]  IParamMin=[]  IParamMax=[]  DParamMin=[]  DParamMax=[]  NParamMin=[]  NParamMax=[]  KbParamMin=[]  KbParamMax=[]  KtParamMin=[]  KtParamMax=[]  KbOutMin=[]  KbOutMax=[]  KtOutMin=[]  KtOutMax=[]  IntegratorOutMin=[]  IntegratorOutMax=[]  FilterOutMin=[]  FilterOutMax=[]  SumI1OutMin=[]  SumI1OutMax=[]  SumI2OutMin=[]  SumI2OutMax=[]  SumI3OutMin=[]  SumI3OutMax=[]  SumI4OutMin=[]  SumI4OutMax=[]  SumDOutMin=[]  SumDOutMax=[]  DifferentiatorOutMin=[]  DifferentiatorOutMax=[]  FilterDiffOutCoefMin=[]  FilterDiffOutCoefMax=[]  ReciprocalOutMin=[]  ReciprocalOutMax=[]  SumDenOutMin=[]  SumDenOutMax=[]  SumNumOutMin=[]  SumNumOutMax=[]  DivideOutMin=[]  DivideOutMax=[]  UdiffTsProdOutMin=[]  UdiffTsProdOutMax=[]  NTsProdOutMin=[]  NTsProdOutMax=[]  UintegralTsProdOutMin=[]  UintegralTsProdOutMax=[]  UngainTsProdOutMin=[]  UngainTsProdOutMax=[]  ClampingZeroOutDataTypeStr=Inherit: Inherit via back propagation  ClampingZeroOutMin=[]  ClampingZeroOutMax=[]  FilterDenConstantOutDataTypeStr=Inherit: Inherit via back propagation  FilterDenConstantOutMin=[]  FilterDenConstantOutMax=[]  PCopyOutDataTypeStr=Inherit: Inherit via back propagation  PCopyOutMin=[]  PCopyOutMax=[]  NCopyOutDataTypeStr=Inherit: Inherit via back propagation  NCopyOutMin=[]  NCopyOutMax=[]  IntegratorContinuousStateAttributes=''  IntegratorStateMustResolveToSignalObject=off  IntegratorRTWStateStorageClass=Auto  FilterContinuousStateAttributes=''  FilterStateMustResolveToSignalObject=off  FilterRTWStateStorageClass=Auto  ParallelPVariant=InternalParameters  IdealPVariant=Disabled  IVariant=InternalParameters  DVariant=Disabled  IntegratorVariant=Discrete  SatVariant=Enabled  AWVariant=DiscClampingParallel  PCopyVariant=Disabled  TRVariant=Disabled  FdbkBlocksVariant=Forward  IdealPFdbkVariant=Disabled  SatFdbkVariant=Disabled  DerivativeFilterVariant=Disabled  NVariant=Disabled  NCopyVariant=Disabled_SignalSpec  FilterICVariant=Disabled  IntegratorICVariant=InternalICs  ExternalResetVariant=Disabled  TRSumVariant=Passthrough  SumFdbkVariant=Disabled  SumVariant=Sum_PI  TsampFilterVariant=InternalTs  TsampNgainVariant=Passthrough  TsampIntegralVariant=Disabled_SignalSpec  ExternalSaturationOutDataTypeStr=Inherit: Same as second input
  PID Controller2 : slpidlib/PID Controller  Controller=PI  Form=Parallel  TimeDomain=Discrete-time  UseExternalTs=off  SampleTime=Ts_Control  IntegratorMethod=Forward Euler  FilterMethod=Forward Euler  ControllerParametersSource=internal  P=Kp_Edq*50  I=Kp_Edq*2*pi*0.01  UseKiTs=off  D=0  N=100  UseFilter=on  TunerSelectOption=Transfer Function Based (PID Tuner App)  InitialConditionSource=internal  InitialConditionForIntegrator=0  InitialConditionForFilter=0  DifferentiatorICPrevScaledInput=0  ExternalReset=none  TrackingMode=off  Kt=1  LimitOutput=on  SatLimitsSource=internal  UpperSaturationLimit=6  LowerSaturationLimit=-6  LinearizeAsGain=on  AntiWindupMode=clamping  Kb=1  LimitIntegrator=off  UpperIntegratorSaturationLimit=inf  LowerIntegratorSaturationLimit=-inf  POutMin=[]  POutMax=[]  IOutMin=[]  IOutMax=[]  DOutMin=[]  DOutMax=[]  NOutMin=[]  NOutMax=[]  SumOutMin=[]  SumOutMax=[]  SaturationOutMin=[]  SaturationOutMax=[]  PParamMin=[]  PParamMax=[]  IParamMin=[]  IParamMax=[]  DParamMin=[]  DParamMax=[]  NParamMin=[]  NParamMax=[]  KbParamMin=[]  KbParamMax=[]  KtParamMin=[]  KtParamMax=[]  KbOutMin=[]  KbOutMax=[]  KtOutMin=[]  KtOutMax=[]  IntegratorOutMin=[]  IntegratorOutMax=[]  FilterOutMin=[]  FilterOutMax=[]  SumI1OutMin=[]  SumI1OutMax=[]  SumI2OutMin=[]  SumI2OutMax=[]  SumI3OutMin=[]  SumI3OutMax=[]  SumI4OutMin=[]  SumI4OutMax=[]  SumDOutMin=[]  SumDOutMax=[]  DifferentiatorOutMin=[]  DifferentiatorOutMax=[]  FilterDiffOutCoefMin=[]  FilterDiffOutCoefMax=[]  ReciprocalOutMin=[]  ReciprocalOutMax=[]  SumDenOutMin=[]  SumDenOutMax=[]  SumNumOutMin=[]  SumNumOutMax=[]  DivideOutMin=[]  DivideOutMax=[]  UdiffTsProdOutMin=[]  UdiffTsProdOutMax=[]  NTsProdOutMin=[]  NTsProdOutMax=[]  UintegralTsProdOutMin=[]  UintegralTsProdOutMax=[]  UngainTsProdOutMin=[]  UngainTsProdOutMax=[]  ClampingZeroOutDataTypeStr=Inherit: Inherit via back propagation  ClampingZeroOutMin=[]  ClampingZeroOutMax=[]  FilterDenConstantOutDataTypeStr=Inherit: Inherit via back propagation  FilterDenConstantOutMin=[]  FilterDenConstantOutMax=[]  PCopyOutDataTypeStr=Inherit: Inherit via back propagation  PCopyOutMin=[]  PCopyOutMax=[]  NCopyOutDataTypeStr=Inherit: Inherit via back propagation  NCopyOutMin=[]  NCopyOutMax=[]  IntegratorContinuousStateAttributes=''  IntegratorStateMustResolveToSignalObject=off  IntegratorRTWStateStorageClass=Auto  FilterContinuousStateAttributes=''  FilterStateMustResolveToSignalObject=off  FilterRTWStateStorageClass=Auto  ParallelPVariant=InternalParameters  IdealPVariant=Disabled  IVariant=InternalParameters  DVariant=Disabled  IntegratorVariant=Discrete  SatVariant=Enabled  AWVariant=DiscClampingParallel  PCopyVariant=Disabled  TRVariant=Disabled  FdbkBlocksVariant=Forward  IdealPFdbkVariant=Disabled  SatFdbkVariant=Disabled  DerivativeFilterVariant=Disabled  NVariant=Disabled  NCopyVariant=Disabled_SignalSpec  FilterICVariant=Disabled  IntegratorICVariant=InternalICs  ExternalResetVariant=Disabled  TRSumVariant=Passthrough  SumFdbkVariant=Disabled  SumVariant=Sum_PI  TsampFilterVariant=InternalTs  TsampNgainVariant=Passthrough  TsampIntegralVariant=Disabled_SignalSpec  ExternalSaturationOutDataTypeStr=Inherit: Same as second input
  PLL (3ph) : spsPLL3phLib/PLL (3ph)  Fmin=45  Par_Init=[0, 50]  ParK=[180, 3200, 1]  TcD=1e-4  MaxRateChangeFreq=1  FilterCutOffFreq=25  Ts=Ts_Control  AGC=on
  Selector : Selector  InputPortWidth=3  IndexOptions=Index vector (dialog)  Indices=[2]  OutputSizes=1
  Selector1 : Selector  InputPortWidth=3  IndexOptions=Index vector (dialog)  Indices=[1]  OutputSizes=1
  Terminator : Terminator
  abc to dq0 : spsabctodq0Lib/abc to dq0  Alignment=Aligned with phase A axis
  Delta_Es : Outport
  wires:
  Add1/1 -> PID Controller2/1
  Constant2/1 -> Add2/2
  Add2/1 -> abc to dq0/2
  PLL (3ph)/2 -> Add2/1
  abc to dq0/1 -> Selector1/1, Selector/1
  Selector1/1 -> Add3/1
  Constant3/1 -> Add3/2
  Add3/1 -> PID Controller1/1
  Es/1 -> PLL (3ph)/1
  Mux/1 -> Delta_Es/1
  Ec/1 -> abc to dq0/1
  Selector/1 -> Add1/1
  Constant1/1 -> Add1/2
  PID Controller1/1 -> Mux/2
  PLL (3ph)/1 -> Terminator/1
  PID Controller2/1 -> Mux/1

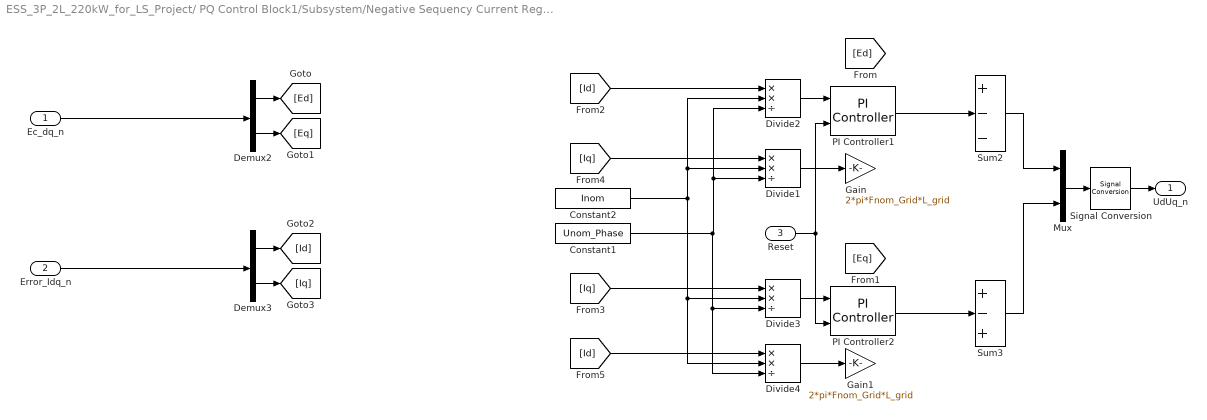
== system ESS_3P_2L_220kW_for_LS_Project/ PQ Control Block1/Subsystem/Negative Sequency Current Regulator ==
  Ec_dq_n : Inport
  Error_Idq_n : Inport  Port=2
  Reset : Inport  Port=3  OutDataTypeStr=boolean
  Constant1 : Constant  Value=Unom_Phase  OutDataTypeStr=Inherit: Inherit via back propagation  SampleTime=-1
  Constant2 : Constant  Value=Inom  OutDataTypeStr=Inherit: Inherit via back propagation  SampleTime=-1
  Demux2 : Demux  Outputs=2
  Demux3 : Demux  Outputs=2
  Divide{1..4} (4 alike) : Product  Inputs=**/  OutDataTypeStr=single
  Gain : Gain  Gain=2*pi*Fnom_Grid*L_grid  ParamDataTypeStr=Inherit: Same as input
  Gain1 : Gain  Gain=2*pi*Fnom_Grid*L_grid  ParamDataTypeStr=Inherit: Same as input
  Mux : Mux  Inputs=2
  PI Controller1 : LibraryForCodeGeneration/PI Controller  Kp=Kp_Idq  Ki=Ki_Idq  Ts=Ts_Control  Max=2  Min=-2
  PI Controller2 : LibraryForCodeGeneration/PI Controller  Kp=Kp_Idq  Ki=Ki_Idq  Ts=Ts_Control  Max=2  Min=-2
  Signal Conversion : SignalConversion  OverrideOpt=off
  Sum2 : Sum  Inputs=+--  InputSameDT=on  SaturateOnIntegerOverflow=on  OutDataTypeStr=Inherit: Same as first input
  Sum3 : Sum  Inputs=+-+  InputSameDT=on  SaturateOnIntegerOverflow=on  OutDataTypeStr=Inherit: Same as first input
  UdUq_n : Outport
  wires:
  [Id] -> Divide4/1
  [Iq] -> Divide1/1
  [Id] -> Divide2/1
  Error_Idq_n/1 -> Demux3/1
  Demux3/1 -> [Id]
  Demux3/2 -> [Iq]
  Demux2/2 -> [Eq]
  Demux2/1 -> [Ed]
  Divide3/1 -> PI Controller2/1
  Mux/1 -> Signal Conversion/1
  Sum2/1 -> Mux/1
  Divide2/1 -> PI Controller1/1
  Sum3/1 -> Mux/2
  Reset/1 -> PI Controller2/2, PI Controller1/2
  Divide1/1 -> Gain/1
  Divide4/1 -> Gain1/1
  Constant2/1 -> Divide1/2, Divide2/2, Divide4/2, Divide3/2
  Constant1/1 -> Divide3/3, Divide4/3, Divide1/3, Divide2/3
  PI Controller2/1 -> Sum3/2
  PI Controller1/1 -> Sum2/2
  Ec_dq_n/1 -> Demux2/1
  Signal Conversion/1 -> UdUq_n/1
  [Iq] -> Divide3/1

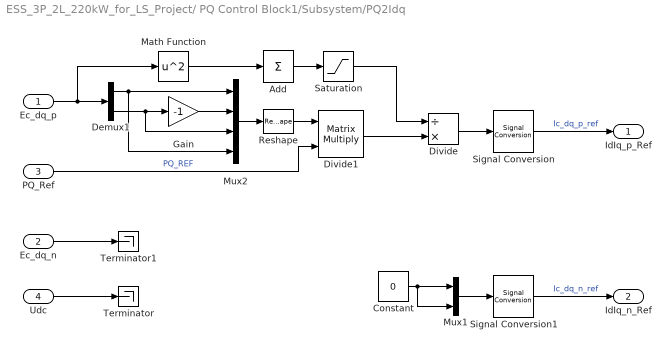
== system ESS_3P_2L_220kW_for_LS_Project/ PQ Control Block1/Subsystem/PQ2Idq ==
  Ec_dq_p : Inport
  Ec_dq_n : Inport  Port=2
  PQ_Ref : Inport  Port=3
  Udc : Inport  Port=4
  Add : Sum  Inputs=+
  Constant : Constant  Value=0  OutDataTypeStr=Inherit: Inherit via back propagation  SampleTime=-1
  Demux1 : Demux  Outputs=2
  Divide : Product  Inputs=/*
  Divide1 : Product  Inputs=**  Multiplication=Matrix(*)
  Gain : Gain  Gain=-1
  Math Function : Math  Operator=square  OutMin=[0.5]  OutMax=[2]
  Mux1 : Mux  Inputs=2
  Mux2 : Mux
  Reshape : Reshape  OutputDimensionality=Customize  OutputDimensions=[2,2]
  Saturation : Saturate  UpperLimit=1.5  LowerLimit=0.5
  Signal Conversion : SignalConversion  OverrideOpt=off
  Signal Conversion1 : SignalConversion  OverrideOpt=off
  Terminator : Terminator
  Terminator1 : Terminator
  IdIq_p_Ref : Outport
  IdIq_n_Ref : Outport  Port=2
  wires:
  Mux1/1 -> Signal Conversion1/1
  PQ_Ref/1 -> Divide1/2  "PQ_REF"
  Signal Conversion/1 -> IdIq_p_Ref/1  "Ic_dq_p_ref"
  Signal Conversion1/1 -> IdIq_n_Ref/1  "Ic_dq_n_ref"
  Constant/1 -> Mux1/2, Mux1/1
  Ec_dq_p/1 -> Math Function/1, Demux1/1
  Udc/1 -> Terminator/1
  Ec_dq_n/1 -> Terminator1/1
  Divide/1 -> Signal Conversion/1
  Demux1/1 -> Mux2/4, Mux2/1
  Gain/1 -> Mux2/2
  Demux1/2 -> Gain/1, Mux2/3
  Mux2/1 -> Reshape/1
  Divide1/1 -> Divide/2
  Reshape/1 -> Divide1/1
  Math Function/1 -> Add/1
  Add/1 -> Saturation/1
  Saturation/1 -> Divide/1

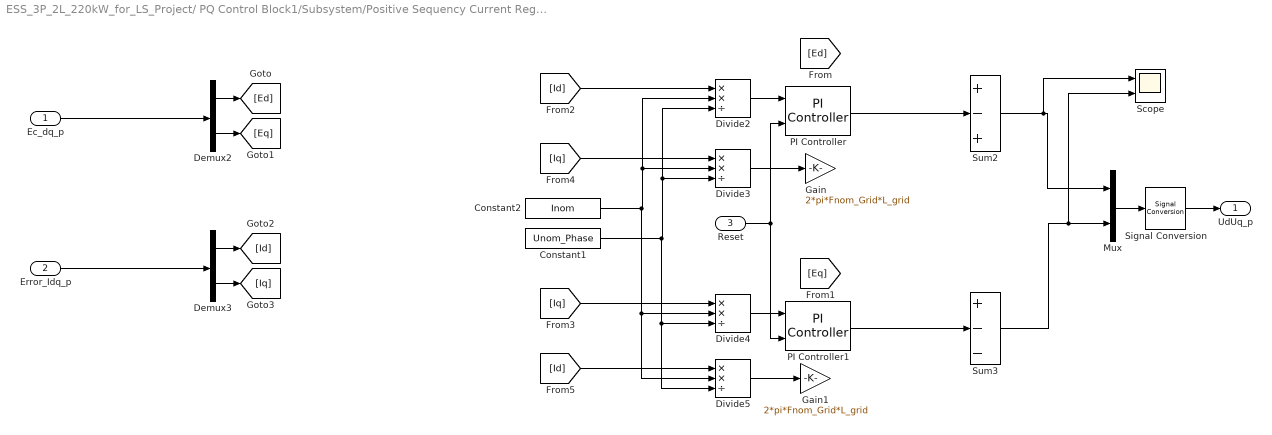
== system ESS_3P_2L_220kW_for_LS_Project/ PQ Control Block1/Subsystem/Positive Sequency Current Regulator ==
  Ec_dq_p : Inport
  Error_Idq_p : Inport  Port=2
  Reset : Inport  Port=3  OutDataTypeStr=boolean
  Constant1 : Constant  Value=Unom_Phase  OutDataTypeStr=Inherit: Inherit via back propagation  SampleTime=-1
  Constant2 : Constant  Value=Inom  OutDataTypeStr=Inherit: Inherit via back propagation  SampleTime=-1
  Demux2 : Demux  Outputs=2
  Demux3 : Demux  Outputs=2
  Divide{2..5} (4 alike) : Product  Inputs=**/  OutDataTypeStr=single
  Gain : Gain  Gain=2*pi*Fnom_Grid*L_grid  ParamDataTypeStr=Inherit: Same as input
  Gain1 : Gain  Gain=2*pi*Fnom_Grid*L_grid  ParamDataTypeStr=Inherit: Same as input
  Mux : Mux  Inputs=2
  PI Controller : LibraryForCodeGeneration/PI Controller  Kp=Kp_Idq  Ki=Ki_Idq  Ts=Ts_Control  Max=2  Min=-2
  PI Controller1 : LibraryForCodeGeneration/PI Controller  Kp=Kp_Idq  Ki=Ki_Idq  Ts=Ts_Control  Max=2  Min=-2
  Scope : Scope  NumInputPorts=2
  Signal Conversion : SignalConversion  OverrideOpt=off
  Sum2 : Sum  Inputs=+-+  InputSameDT=on  SaturateOnIntegerOverflow=on  OutDataTypeStr=Inherit: Same as first input
  Sum3 : Sum  Inputs=+--  InputSameDT=on  SaturateOnIntegerOverflow=on  OutDataTypeStr=Inherit: Same as first input
  UdUq_p : Outport
  wires:
  [Iq] -> Divide4/1
  Sum2/1 -> Scope/1, Mux/1
  Divide3/1 -> Gain/1
  Divide5/1 -> Gain1/1
  [Id] -> Divide2/1
  Divide4/1 -> PI Controller1/1
  Demux2/1 -> [Ed]
  Demux2/2 -> [Eq]
  Demux3/2 -> [Iq]
  Demux3/1 -> [Id]
  Error_Idq_p/1 -> Demux3/1
  [Iq] -> Divide3/1
  [Id] -> Divide5/1
  PI Controller/1 -> Sum2/2
  Divide2/1 -> PI Controller/1
  Reset/1 -> PI Controller1/2, PI Controller/2
  Constant2/1 -> Divide5/2, Divide4/2, Divide3/2, Divide2/2
  Constant1/1 -> Divide5/3, Divide4/3, Divide3/3, Divide2/3
  PI Controller1/1 -> Sum3/2
  Ec_dq_p/1 -> Demux2/1
  Mux/1 -> Signal Conversion/1
  Signal Conversion/1 -> UdUq_p/1
  Sum3/1 -> Scope/2, Mux/2

== system ESS_3P_2L_220kW_for_LS_Project/ PQ Control Block1/Subsystem/Ref2Error ==
  "Ic_ABC " : Inport
  "IdIq_p_Ref " : Inport  Port=2
  IdIq_n_Ref : Inport  Port=3
  wt : Inport  Port=4
  Add : Sum  Inputs=-++
  Gain : Gain  Gain=-1
  Scope : Scope  NumInputPorts=2
  Selector : Selector  InputPortWidth=3  IndexOptions=Index vector (dialog)  Indices=[1 2]  OutputSizes=1
  Signal Conversion : SignalConversion  OverrideOpt=off
  Signal Conversion1 : SignalConversion  OverrideOpt=off
  abc2αβ0 : LibraryForCodeGeneration/abc2αβ0  SystemSampleTime=-1  VariantActivationTime=update diagram  AllowFlexibleInterface=on  Latency=0  AutoFrameSizeCalculation=off
  dq2αβ0 : LibraryForCodeGeneration/dq2αβ  SystemSampleTime=-1  VariantActivationTime=update diagram  AllowFlexibleInterface=on  Latency=0  AutoFrameSizeCalculation=off
  dq2αβ1 : LibraryForCodeGeneration/dq2αβ  SystemSampleTime=-1  VariantActivationTime=update diagram  AllowFlexibleInterface=on  Latency=0  AutoFrameSizeCalculation=off
  αβ2dq : LibraryForCodeGeneration/αβ2dq  SystemSampleTime=-1  VariantActivationTime=update diagram  AllowFlexibleInterface=on  Latency=0  AutoFrameSizeCalculation=off
  αβ2dq1 : LibraryForCodeGeneration/αβ2dq  SystemSampleTime=-1  VariantActivationTime=update diagram  AllowFlexibleInterface=on  Latency=0  AutoFrameSizeCalculation=off
  Error_Idq_p : Outport
  Error_Idq_n : Outport  Port=2
  wires:
  "Ic_ABC "/1 -> abc2αβ0/1
  αβ2dq/1 -> Scope/1, Signal Conversion/1
  αβ2dq1/1 -> Scope/2, Signal Conversion1/1
  wt/1 -> dq2αβ0/2, αβ2dq/2, Gain/1
  abc2αβ0/1 -> Selector/1
  "IdIq_p_Ref "/1 -> dq2αβ0/1
  Gain/1 -> dq2αβ1/2, αβ2dq1/2
  IdIq_n_Ref/1 -> dq2αβ1/1
  dq2αβ0/1 -> Add/2
  dq2αβ1/1 -> Add/3
  Selector/1 -> Add/1
  Add/1 -> αβ2dq1/1, αβ2dq/1
  Signal Conversion/1 -> Error_Idq_p/1
  Signal Conversion1/1 -> Error_Idq_n/1

== system ESS_3P_2L_220kW_for_LS_Project/ PQ Control Block1/Subsystem/Udq2Uabc ==
  Udq_p : Inport
  Udq_n : Inport  Port=2
  Udc : Inport  Port=3
  wt : Inport  Port=4
  Add : Sum
  Constant : Constant  Value=2*sqrt(2)  OutDataTypeStr=Inherit: Inherit via back propagation  SampleTime=-1
  Constant3 : Constant  Value=Unom_Phase  OutDataTypeStr=Inherit: Inherit via back propagation  SampleTime=-1
  Constant6 : Constant  Value=Udc_ref  OutDataTypeStr=Inherit: Inherit via back propagation  SampleTime=-1
  Divide : Product  Inputs=***//  OutDataTypeStr=single
  Gain2 : Gain  Gain=-1  ParamDataTypeStr=Inherit: Same as input
  dq2abc : LibraryForCodeGeneration/dq2abc  SystemSampleTime=-1  VariantActivationTime=update diagram  AllowFlexibleInterface=on  Latency=0  AutoFrameSizeCalculation=off
  dq2abc1 : LibraryForCodeGeneration/dq2abc  SystemSampleTime=-1  VariantActivationTime=update diagram  AllowFlexibleInterface=on  Latency=0  AutoFrameSizeCalculation=off
  Uabc : Outport
  wires:
  dq2abc1/1 -> Add/2
  wt/1 -> dq2abc/2, Gain2/1
  Udq_p/1 -> dq2abc/1
  Udq_n/1 -> dq2abc1/1
  dq2abc/1 -> Add/1
  Constant6/1 -> Divide/5
  Constant/1 -> Divide/3
  Constant3/1 -> Divide/2
  Add/1 -> Divide/1
  Udc/1 -> Divide/4
  Divide/1 -> Uabc/1
  Gain2/1 -> dq2abc1/2
